simulink model "ActualDroneSetup"  (R2025a)
settings: Solver=VariableStepAuto  StartTime=0.0  StopTime=10.0  RelTol=1e-3
InitFcn:
  | %% System Constants
  | 
  | % mass
  | m = 0.12635;
  | 
  | % graviational constant
  | g = 9.81;
  | 
  | % Moment of inertia
  | I_XX = 0.00016159;
  | I_YY = 0.00016466;
  | I_ZZ = 0.00026144;
  | 
  | % thrust and power factor - needs to be measured
  | c_t = 1;
  | c_p = 1;
  | 
  | % https://en.wikipedia.org/wiki/Density_of_air
  | rho = 1.225;
  | 
  | % surface area of a propeller - estimation based on half of circle area
  | diameter = 0.04;
  | A = pi * (diameter/2)^2 / 2;
  | 
  | % chord length - needs to be measured
  | r = 0.008;
  | 
  | %Thrust coefficient
  | b = c_t * rho * A * r^2;
  | 
  | %Torque drag coefficient
  | d_t = c_p * rho * A * r^3;
  | 
  | %Distance from CoG to propeller axis
  | l = 0.104707;
libraries: arduinosensorlib x1
settings Model: Creator=tobia  LastModifiedBy=dma

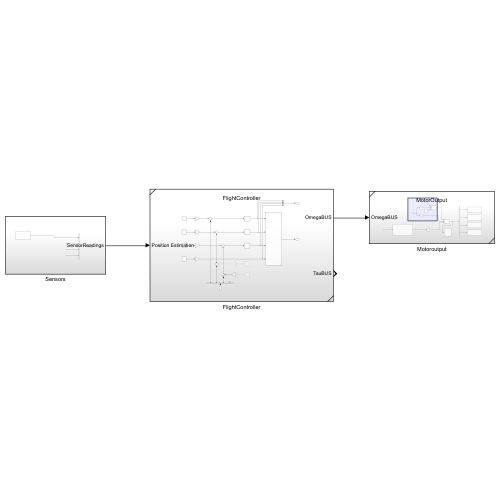
[thumbnail: Simulink's stored preview of the top-level diagram]
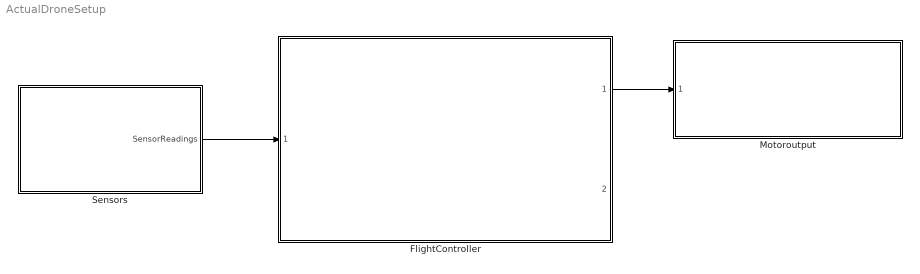
== system ActualDroneSetup ==
  FlightController : Subsystem  ReferencedSubsystem=FlightController
  Motoroutput : Subsystem  ReferencedSubsystem=MotorOutput
  Sensors : Subsystem
  wires:
  Sensors/1(SensorReadings) -> FlightController/1
  FlightController/1 -> Motoroutput/1

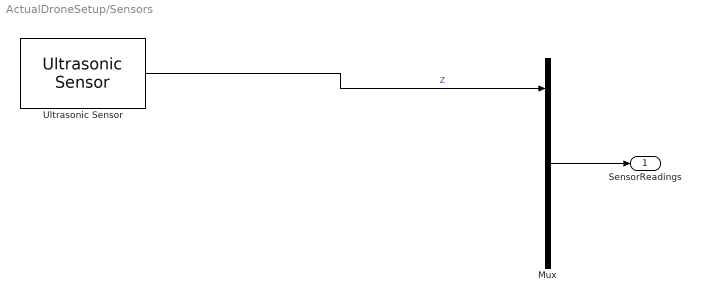
== system ActualDroneSetup/Sensors ==
  Mux : Mux
  Ultrasonic Sensor : arduinosensorlib/Ultrasonic Sensor  NumSignalPins=1  TrigPin=4  EchoPin=5  SignalPin=3  SampleTime_=0.1  blockPlatform=ARDUINO
  SensorReadings : Outport
  wires:
  Mux/1 -> SensorReadings/1
  Ultrasonic Sensor/1 -> Mux/1  "Z"
  ? -> Mux/2  "phi"
  ? -> Mux/3  "theta"
  ? -> Mux/4  "psi"
